simulink model "fxpdemo_sfun_user_const_rtw"  (Simulink 5.0)
settings: Solver=FixedStepDiscrete  StartTime=0.0  StopTime=1  FixedStep=1  RelTol=1e-3
settings Model: Creator=andyb  LastModifiedBy=andyb  ExtModeAutoUpdateStatusClock=off  RTWOptions="-aEnforceIntegerDowncast=1 -aExtMode=0 -aExtModeTesting=0 -aFoldNonRolledExpr=1 -aForceParamTrailComments=0 -aGenerateComments=1 -aGenerateReport=1 -aIgnoreCustomStorageClasses=1 -aIncDataTypeInIds=0 -aIncHierarchyInIds=0 -aInlineInvariantSignals=0 -aInlineParameters=0 -aInlinedPrmAccess=\"Literals\" -aLocalBlockOutputs=1 -aLogVarNameModifier=\"rt_\" -aMaxRTWIdLen=31 -aPrefixModelToSubsysFcnNames=1 -aRTWVerbose=1 -aRollThreshold=5 -aShowEliminatedStatements=0"

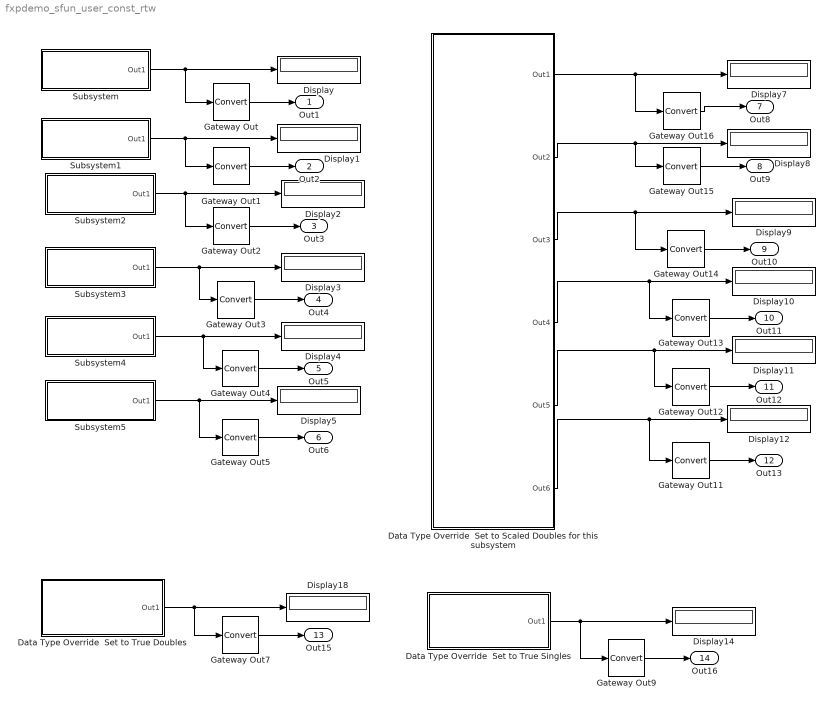
== system fxpdemo_sfun_user_const_rtw ==
  Data Type Override  Set to Scaled Doubles for this subsystem : Subsystem  DataTypeOverride=ScaledDoubles
  Data Type Override  Set to True Doubles : Subsystem  DataTypeOverride=TrueDoubles
  Data Type Override  Set to True Singles : Subsystem  DataTypeOverride=TrueSingles
  Display{,1..5,7..12,14,18} (14 alike) : Display
  Gateway Out{,1..5,7,9,11..16} (14 alike) : DataTypeConversion  DataType=double
  Subsystem : Subsystem  mask{storedInt=33, isSigned=on, numBits=7, numFracBits=2}
      mask prompts: storedInt "Stored Integer Value"; isSigned "Signed integer (otherwise unsigned integer)"; numBits "Total Number of Bits"; numFracBits "Number of Bits to Right of Binary Point"
      mask Display: disp(sprintf('User SFunction\nFixed Point\nConstant'))
  Subsystem1 : Subsystem  mask{storedInt=33, isSigned=on, numBits=12, numFracBits=2}
      mask prompts: storedInt "Stored Integer Value"; isSigned "Signed integer (otherwise unsigned integer)"; numBits "Total Number of Bits"; numFracBits "Number of Bits to Right of Binary Point"
      mask Display: disp(sprintf('User SFunction\nFixed Point\nConstant'))
  Subsystem2 : Subsystem  mask{storedInt=33, isSigned=on, numBits=17, numFracBits=2}
      mask prompts: storedInt "Stored Integer Value"; isSigned "Signed integer (otherwise unsigned integer)"; numBits "Total Number of Bits"; numFracBits "Number of Bits to Right of Binary Point"
      mask Display: disp(sprintf('User SFunction\nFixed Point\nConstant'))
  Subsystem3 : Subsystem  mask{storedInt=33, isSigned=off, numBits=7, numFracBits=2}
      mask prompts: storedInt "Stored Integer Value"; isSigned "Signed integer (otherwise unsigned integer)"; numBits "Total Number of Bits"; numFracBits "Number of Bits to Right of Binary Point"
      mask Display: disp(sprintf('User SFunction\nFixed Point\nConstant'))
  Subsystem4 : Subsystem  mask{storedInt=33, isSigned=off, numBits=12, numFracBits=2}
      mask prompts: storedInt "Stored Integer Value"; isSigned "Signed integer (otherwise unsigned integer)"; numBits "Total Number of Bits"; numFracBits "Number of Bits to Right of Binary Point"
      mask Display: disp(sprintf('User SFunction\nFixed Point\nConstant'))
  Subsystem5 : Subsystem  mask{storedInt=33, isSigned=off, numBits=17, numFracBits=2}
      mask prompts: storedInt "Stored Integer Value"; isSigned "Signed integer (otherwise unsigned integer)"; numBits "Total Number of Bits"; numFracBits "Number of Bits to Right of Binary Point"
      mask Display: disp(sprintf('User SFunction\nFixed Point\nConstant'))
  Out1 : Outport
  Out2 : Outport  Port=2
  Out3 : Outport  Port=3
  Out4 : Outport  Port=4
  Out5 : Outport  Port=5
  Out6 : Outport  Port=6
  Out8 : Outport  Port=7
  Out9 : Outport  Port=8
  Out10 : Outport  Port=9
  Out11 : Outport  Port=10
  Out12 : Outport  Port=11
  Out13 : Outport  Port=12
  Out15 : Outport  Port=13
  Out16 : Outport  Port=14
  wires:
  Subsystem/1(Out1) -> Display/1, Gateway Out/1
  Subsystem1/1(Out1) -> Display1/1, Gateway Out1/1
  Subsystem2/1(Out1) -> Display2/1, Gateway Out2/1
  Subsystem3/1(Out1) -> Display3/1, Gateway Out3/1
  Subsystem4/1(Out1) -> Display4/1, Gateway Out4/1
  Subsystem5/1(Out1) -> Display5/1, Gateway Out5/1
  Gateway Out/1 -> Out1/1
  Gateway Out1/1 -> Out2/1
  Gateway Out2/1 -> Out3/1
  Gateway Out3/1 -> Out4/1
  Gateway Out4/1 -> Out5/1
  Gateway Out5/1 -> Out6/1
  Data Type Override  Set to Scaled Doubles for this subsystem/1(Out1) -> Display7/1, Gateway Out16/1
  Data Type Override  Set to Scaled Doubles for this subsystem/2(Out2) -> Display8/1, Gateway Out15/1
  Data Type Override  Set to Scaled Doubles for this subsystem/3(Out3) -> Display9/1, Gateway Out14/1
  Data Type Override  Set to Scaled Doubles for this subsystem/4(Out4) -> Display10/1, Gateway Out13/1
  Data Type Override  Set to Scaled Doubles for this subsystem/5(Out5) -> Display11/1, Gateway Out12/1
  Data Type Override  Set to Scaled Doubles for this subsystem/6(Out6) -> Display12/1, Gateway Out11/1
  Gateway Out16/1 -> Out8/1
  Gateway Out15/1 -> Out9/1
  Gateway Out14/1 -> Out10/1
  Gateway Out13/1 -> Out11/1
  Gateway Out12/1 -> Out12/1
  Gateway Out11/1 -> Out13/1
  Data Type Override  Set to True Doubles/1(Out1) -> Display18/1, Gateway Out7/1
  Gateway Out7/1 -> Out15/1
  Data Type Override  Set to True Singles/1(Out1) -> Display14/1, Gateway Out9/1
  Gateway Out9/1 -> Out16/1

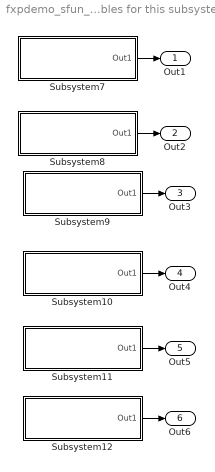
== system fxpdemo_sfun_user_const_rtw/Data Type Override  Set to Scaled Doubles for this subsystem ==
  Subsystem10 : Subsystem  mask{storedInt=33, isSigned=off, numBits=7, numFracBits=2}
      mask prompts: storedInt "Stored Integer Value"; isSigned "Signed integer (otherwise unsigned integer)"; numBits "Total Number of Bits"; numFracBits "Number of Bits to Right of Binary Point"
      mask Display: disp(sprintf('User SFunction\nFixed Point\nConstant'))
  Subsystem11 : Subsystem  mask{storedInt=33, isSigned=off, numBits=12, numFracBits=2}
      mask prompts: storedInt "Stored Integer Value"; isSigned "Signed integer (otherwise unsigned integer)"; numBits "Total Number of Bits"; numFracBits "Number of Bits to Right of Binary Point"
      mask Display: disp(sprintf('User SFunction\nFixed Point\nConstant'))
  Subsystem12 : Subsystem  mask{storedInt=33, isSigned=off, numBits=17, numFracBits=2}
      mask prompts: storedInt "Stored Integer Value"; isSigned "Signed integer (otherwise unsigned integer)"; numBits "Total Number of Bits"; numFracBits "Number of Bits to Right of Binary Point"
      mask Display: disp(sprintf('User SFunction\nFixed Point\nConstant'))
  Subsystem7 : Subsystem  mask{storedInt=33, isSigned=on, numBits=7, numFracBits=2}
      mask prompts: storedInt "Stored Integer Value"; isSigned "Signed integer (otherwise unsigned integer)"; numBits "Total Number of Bits"; numFracBits "Number of Bits to Right of Binary Point"
      mask Display: disp(sprintf('User SFunction\nFixed Point\nConstant'))
  Subsystem8 : Subsystem  mask{storedInt=33, isSigned=on, numBits=12, numFracBits=2}
      mask prompts: storedInt "Stored Integer Value"; isSigned "Signed integer (otherwise unsigned integer)"; numBits "Total Number of Bits"; numFracBits "Number of Bits to Right of Binary Point"
      mask Display: disp(sprintf('User SFunction\nFixed Point\nConstant'))
  Subsystem9 : Subsystem  mask{storedInt=33, isSigned=on, numBits=17, numFracBits=2}
      mask prompts: storedInt "Stored Integer Value"; isSigned "Signed integer (otherwise unsigned integer)"; numBits "Total Number of Bits"; numFracBits "Number of Bits to Right of Binary Point"
      mask Display: disp(sprintf('User SFunction\nFixed Point\nConstant'))
  Out1 : Outport
  Out2 : Outport  Port=2
  Out3 : Outport  Port=3
  Out4 : Outport  Port=4
  Out5 : Outport  Port=5
  Out6 : Outport  Port=6
  wires:
  Subsystem7/1(Out1) -> Out1/1
  Subsystem8/1(Out1) -> Out2/1
  Subsystem9/1(Out1) -> Out3/1
  Subsystem10/1(Out1) -> Out4/1
  Subsystem11/1(Out1) -> Out5/1
  Subsystem12/1(Out1) -> Out6/1

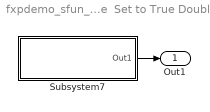
== system fxpdemo_sfun_user_const_rtw/Data Type Override  Set to True Doubles ==
  Subsystem7 : Subsystem  mask{storedInt=33, isSigned=on, numBits=7, numFracBits=2}
      mask prompts: storedInt "Stored Integer Value"; isSigned "Signed integer (otherwise unsigned integer)"; numBits "Total Number of Bits"; numFracBits "Number of Bits to Right of Binary Point"
      mask Display: disp(sprintf('User SFunction\nFixed Point\nConstant'))
  Out1 : Outport
  wires:
  Subsystem7/1(Out1) -> Out1/1

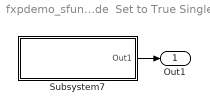
== system fxpdemo_sfun_user_const_rtw/Data Type Override  Set to True Singles ==
  Subsystem7 : Subsystem  mask{storedInt=33, isSigned=on, numBits=7, numFracBits=2}
      mask prompts: storedInt "Stored Integer Value"; isSigned "Signed integer (otherwise unsigned integer)"; numBits "Total Number of Bits"; numFracBits "Number of Bits to Right of Binary Point"
      mask Display: disp(sprintf('User SFunction\nFixed Point\nConstant'))
  Out1 : Outport
  wires:
  Subsystem7/1(Out1) -> Out1/1

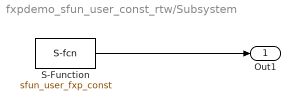
== system fxpdemo_sfun_user_const_rtw/Subsystem ==
  S-Function : S-Function  FunctionName=sfun_user_fxp_const  Parameters=storedInt, isSigned, numBits, numFracBits
  Out1 : Outport
  wires:
  S-Function/1 -> Out1/1

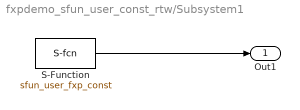
== system fxpdemo_sfun_user_const_rtw/Subsystem1 ==
  S-Function : S-Function  FunctionName=sfun_user_fxp_const  Parameters=storedInt, isSigned, numBits, numFracBits
  Out1 : Outport
  wires:
  S-Function/1 -> Out1/1

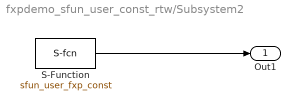
== system fxpdemo_sfun_user_const_rtw/Subsystem2 ==
  S-Function : S-Function  FunctionName=sfun_user_fxp_const  Parameters=storedInt, isSigned, numBits, numFracBits
  Out1 : Outport
  wires:
  S-Function/1 -> Out1/1

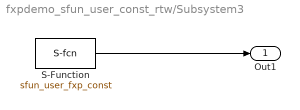
== system fxpdemo_sfun_user_const_rtw/Subsystem3 ==
  S-Function : S-Function  FunctionName=sfun_user_fxp_const  Parameters=storedInt, isSigned, numBits, numFracBits
  Out1 : Outport
  wires:
  S-Function/1 -> Out1/1

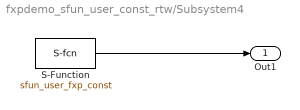
== system fxpdemo_sfun_user_const_rtw/Subsystem4 ==
  S-Function : S-Function  FunctionName=sfun_user_fxp_const  Parameters=storedInt, isSigned, numBits, numFracBits
  Out1 : Outport
  wires:
  S-Function/1 -> Out1/1

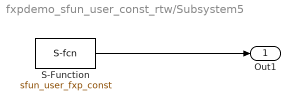
== system fxpdemo_sfun_user_const_rtw/Subsystem5 ==
  S-Function : S-Function  FunctionName=sfun_user_fxp_const  Parameters=storedInt, isSigned, numBits, numFracBits
  Out1 : Outport
  wires:
  S-Function/1 -> Out1/1

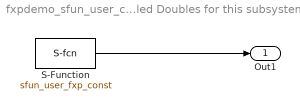
== system fxpdemo_sfun_user_const_rtw/Data Type Override  Set to Scaled Doubles for this subsystem/Subsystem10 ==
  S-Function : S-Function  FunctionName=sfun_user_fxp_const  Parameters=storedInt, isSigned, numBits, numFracBits
  Out1 : Outport
  wires:
  S-Function/1 -> Out1/1

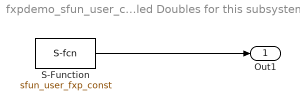
== system fxpdemo_sfun_user_const_rtw/Data Type Override  Set to Scaled Doubles for this subsystem/Subsystem11 ==
  S-Function : S-Function  FunctionName=sfun_user_fxp_const  Parameters=storedInt, isSigned, numBits, numFracBits
  Out1 : Outport
  wires:
  S-Function/1 -> Out1/1

== system fxpdemo_sfun_user_const_rtw/Data Type Override  Set to Scaled Doubles for this subsystem/Subsystem12 ==
  S-Function : S-Function  FunctionName=sfun_user_fxp_const  Parameters=storedInt, isSigned, numBits, numFracBits
  Out1 : Outport
  wires:
  S-Function/1 -> Out1/1

== system fxpdemo_sfun_user_const_rtw/Data Type Override  Set to Scaled Doubles for this subsystem/Subsystem7 ==
  S-Function : S-Function  FunctionName=sfun_user_fxp_const  Parameters=storedInt, isSigned, numBits, numFracBits
  Out1 : Outport
  wires:
  S-Function/1 -> Out1/1

== system fxpdemo_sfun_user_const_rtw/Data Type Override  Set to Scaled Doubles for this subsystem/Subsystem8 ==
  S-Function : S-Function  FunctionName=sfun_user_fxp_const  Parameters=storedInt, isSigned, numBits, numFracBits
  Out1 : Outport
  wires:
  S-Function/1 -> Out1/1

== system fxpdemo_sfun_user_const_rtw/Data Type Override  Set to Scaled Doubles for this subsystem/Subsystem9 ==
  S-Function : S-Function  FunctionName=sfun_user_fxp_const  Parameters=storedInt, isSigned, numBits, numFracBits
  Out1 : Outport
  wires:
  S-Function/1 -> Out1/1

== system fxpdemo_sfun_user_const_rtw/Data Type Override  Set to True Doubles/Subsystem7 ==
  S-Function : S-Function  FunctionName=sfun_user_fxp_const  Parameters=storedInt, isSigned, numBits, numFracBits
  Out1 : Outport
  wires:
  S-Function/1 -> Out1/1

== system fxpdemo_sfun_user_const_rtw/Data Type Override  Set to True Singles/Subsystem7 ==
  S-Function : S-Function  FunctionName=sfun_user_fxp_const  Parameters=storedInt, isSigned, numBits, numFracBits
  Out1 : Outport
  wires:
  S-Function/1 -> Out1/1
